simulink model "pid_ramp"  (R2018b)
settings: Solver=FixedStepAuto  StartTime=0.0  StopTime=10  FixedStep=0.001  RelTol=0.005
values from neighbouring files (symbols this model uses):
  A = [-b/J   K/J ... (first row only)    [motor_model.m]
  B = [0 ... (first row only)    [motor_model.m]
  C = [1   0]    [motor_model.m]
  D = 0    [motor_model.m]
settings Model: Creator=kika  LastModifiedBy=kika
settings DataIOCC: ReturnWorkspaceOutputs=on

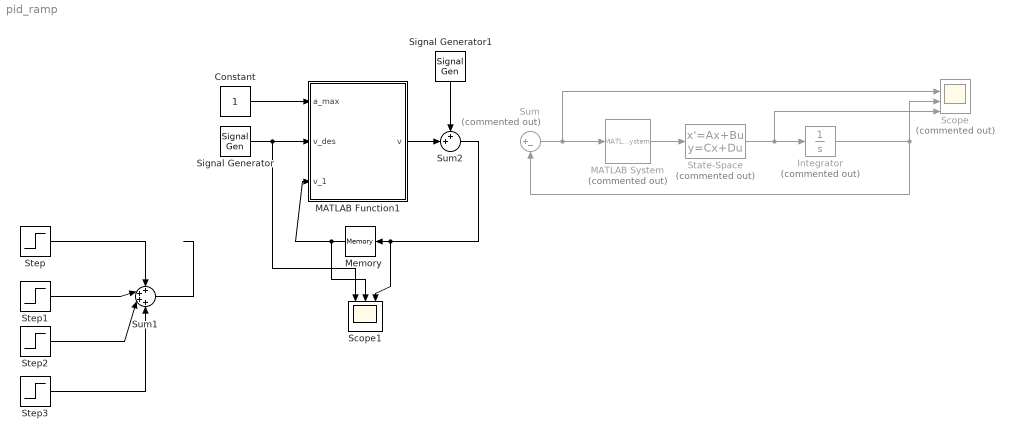
== system pid_ramp ==
  Constant : Constant
  Integrator : Integrator  Commented=on
  MATLAB Function1 : MATLAB Function  TreatAsAtomicUnit=on
  MATLAB System : MATLABSystem  Commented=on  System=PID  kp=10  ki=0  kd=0  dt=0.0005  kt=0  u_max=10  u_min=-10  SimulateUsing=Interpreted execution
      mask Type: PID
      mask Display:
      | disp('PID');
      | port_label('input',1,'e');
      | port_label('output',1,'y');
  Memory : Memory
  Scope : Scope  Commented=on  NumInputPorts=4
  Scope1 : Scope  NumInputPorts=3
  Signal Generator : SignalGenerator  Frequency=5  Units=rad/sec
  Signal Generator1 : SignalGenerator  WaveForm=random  Amplitude=0.001  Frequency=10  Units=rad/sec
  State-Space : StateSpace  Commented=on  A=A  B=B  C=C  D=D  InitialCondition=[0,0]'
  Step : Step  SampleTime=0
  Step1 : Step  Time=2  After=-1  SampleTime=0
  Step2 : Step  Time=3  After=-2  SampleTime=0
  Step3 : Step  Time=3  After=-2  SampleTime=0
  Sum : Sum  Commented=on  Inputs=|+-
  Sum1 : Sum  Inputs=++++
  Sum2 : Sum  Inputs=++|
  wires:
  MATLAB System/1 -> State-Space/1
  Sum/1 -> Scope/2, MATLAB System/1
  State-Space/1 -> Scope/4, Integrator/1
  Integrator/1 -> Sum/2, Scope/3
  Sum2/1 -> Scope1/3, Memory/1
  Memory/1 -> Scope1/2, MATLAB Function1/3(v_1)
  Sum1/1 -> ?
  Constant/1 -> MATLAB Function1/1(a_max)
  Step/1 -> Sum1/1
  Step1/1 -> Sum1/2
  Step2/1 -> Sum1/3
  Step3/1 -> Sum1/4
  Signal Generator/1 -> MATLAB Function1/2(v_des), Scope1/1
  MATLAB Function1/1(v) -> Sum2/2
  Signal Generator1/1 -> Sum2/1

== matlab function pid_ramp/MATLAB Function1 ==
  data: a_max input; v output size=[1,1]; v_des input; v_1 input
function v = ramp(a_max, v_des, v_1)

    dt = 0.001;
    
    direction = 0;
    if (v_des - v_1) > eps
        direction = 1;
    elseif (v_des - v_1) < -eps
        direction = -1;
    end
    
    v = v_1 + direction * a_max * dt;
    
%     if v_1 >= v_des
%         v = v_des;
%     elseif v_1 <= v_des
%         v = -v_des;
%     end
